simulink model "MR_CIGRE_GENERALIZADO"  (R2017b)
settings: Solver=ode23tb  StartTime=0.0  StopTime=t_sim  RelTol=1e-4
values from neighbouring files (symbols this model uses):
  BAT1_CONT = 0    [Dados_MR_CIGRE_generalizado.m]
  BAT2_CONT = 0    [Dados_MR_CIGRE_generalizado.m]
  Cdc = 19.24E-6/2    (= 9.62e-06)    [Dados_de_Intermit.m]    (also in Dados_de_Intermit_old.m)
  Cf = 5E-6    (= 5e-06)    [Dados_de_Intermit.m]    (also in Dados_de_Intermit_old.m)
  f0 = 50    [Dados_MR_CIGRE_generalizado.m]
  Imax_solar1 = 1.5 * I_nom_solar1 * sqrt(2)    [Dados_de_Intermit.m]
  Imax_solar2 = 1.5 * I_nom_solar2 * sqrt(2)    [Dados_de_Intermit.m]
  Ki_interm = (R+ron)/ti    (= 201.76)    [Dados_de_Intermit.m]
  Kp_cp = 0.2    [Dados_de_Intermit.m]
  Kp_cr = 0.4e-3    (= 0.0004)    [Dados_de_Intermit.m]
  Kp_interm = L/ti    (= 2.7)    [Dados_de_Intermit.m]
  L = 1.35E-3    (= 0.00135)    [Dados_de_Intermit.m]    (also in Dados_de_Intermit_old.m)
  LPF_P_Interm = 100    [Dados_de_Intermit.m]
  P_Solar1 = 21e3    (= 21000)    [Dados_MR_CIGRE_generalizado.m]
  P_Solar2 = 21e3    (= 21000)    [Dados_MR_CIGRE_generalizado.m]
  PQ_ref_time_bat1 = t_estab    (= 1)    [Dados_MR_CIGRE_generalizado.m]
  Pref_Bat1 = 0*1e3    (= 0)    [Dados_MR_CIGRE_generalizado.m]
  Qref_Bat1 = 0*1e3    (= 0)    [Dados_MR_CIGRE_generalizado.m]
  Qref_Solar = 0    [Dados_MR_CIGRE_generalizado.m]
  R = 0.1    [Dados_de_Intermit.m]    (also in Dados_de_Intermit_old.m)
  ron = 0.88E-3    (= 0.00088)    [Dados_de_Intermit.m]    (also in Dados_de_Intermit_old.m)
  Sb_Bat1 = 45e3    (= 45000)    [Dados_MR_CIGRE_generalizado.m]
  Sb_sol1 = 20e3    (= 20000)    [Dados_MR_CIGRE_generalizado.m]
  Sb_sol2 = 20e3    (= 20000)    [Dados_MR_CIGRE_generalizado.m]
  t_atraso = 0    [Dados_MR_CIGRE_generalizado.m]
  theta1 = 45*rad    (= 0.785398163397)    [Dados_MR_CIGRE_generalizado.m]
  theta2 = 45*rad    (= 0.785398163397)    [Dados_MR_CIGRE_generalizado.m]
  ti_cp = 10e-3    (= 0.01)    [Dados_de_Intermit.m]
  ti_cr = 10e-3    (= 0.01)    [Dados_de_Intermit.m]
  tilha = 0.6    [Dados_MR_CIGRE_generalizado.m]
  tsinc = 6    [Dados_MR_CIGRE_generalizado.m]
  Vdc = 700    [Dados_de_Intermit.m]    (also in Dados_de_Intermit_old.m)
  Vs1 = 20000    [Dados_MR_CIGRE_generalizado.m]
  Vs2 = 400    [Dados_MR_CIGRE_generalizado.m]
  w0 = 2*pi*f0    (= 314.159265359)    [Dados_MR_CIGRE_generalizado.m]
undefined symbols (not defined in the file or in its folder): Cdc_Bat1, Cf_Bat1, cont_fre, cont_ten, I_max_Bat1, Is_bat1, K_iff_Bat1, Kcij, Ki_Bat1, Kie, Kiw, Kp_Bat1, Kpe, Kpw, Kv_Bat1, Kvi_DC, Kvp_DC, L_10_18, L_12_13, L_13_14, L_14_15, L_1_2, L_2_3, L_3_11, L_3_4, L_4_12, L_4_5, L_5_6, L_6_16, L_6_7, L_7_8, L_8_9, L_9_10, L_9_17, L_Bat1, L_Bat2, L_Virt_Bat1, L_Virt_Bat2, LC_Bat2, Lfsj, LPF_Ci_Bat1, LPF_Ci_Bat2, LPF_Cv_Bat1, LPF_P_Bat1, LPF_Q_Bat1, LPF_Vdc, m_Bat1, n_Bat1, PQ_ref_taxavar_bat1, R_10_18, R_12_13, R_13_14, R_14_15, R_1_2, R_2_3, R_3_11, R_3_4, R_4_12, R_4_5, R_5_6 ... (+32)
libraries: powerlib x158, powerlib_meascontrol x59, re_lib x2, simulink x1
(part 3 of 4)

== system MR_CIGRE_GENERALIZADO/Banco de Baterias_1/Bateria e Conversor CC//CC ==
  note: Bateria
  note: Conversor CC e chopper
  note: Medidas Bateria
  D : Inport
  CM2 : powerlib/Measurements/Current Measurement  PhasorSimulation=off  OutputType=Complex  PSBequivalent=0
  DC Voltage Source : powerlib/Electrical Sources/DC Voltage Source  Amplitude=Voc_bat1  Measurements=None
  P : Product  Inputs=**
  Series RLC Branch : powerlib/Elements/Series RLC Branch  LConnTagsString=__new0  RConnTagsString=__new0  BranchType=RL  Resistance=Rfsj  Inductance=Lfsj  SetiL0=on  InitialCurrent=0  Capacitance=1e-6  Setx0=off  InitialVoltage=0  Measurements=None
  Series RLC Branch1 : powerlib/Elements/Series RLC Branch  LConnTagsString=__new0  RConnTagsString=__new0  BranchType=R  Resistance=Rb_bat1  Inductance=1e-3  SetiL0=off  InitialCurrent=0  Capacitance=1e-6  Setx0=off  InitialVoltage=0  Measurements=None
  Two-Quadrant DC/DC Converter : powerlib/Power Electronics/Two-Quadrant DC//DC Converter  ModelType=Average model (D-controlled)  Ron=1e-3  Rs=1e6  Cs=inf  Vforward=[0,0]  Ron_Diode=1e-3  Rs_Diode=1e6  Cs_Diode=inf  Vf_Diode=1e-3  Rs_CurrentSource=inf
      settings: SourceProductName=Simscape Power Systems  SourceProductBaseCode=PS
  VM2 : powerlib/Measurements/Voltage Measurement  PhasorSimulation=off  OutputType=Complex  PSBequivalent=0
  + out : PMIOPort  Port=1  Side=Left
  - out : PMIOPort  Port=2  Side=Left
  Ibat : Outport
  Vbat : Outport  Port=2
  Pbat : Outport  Port=3
  wires:
  CM2/1 -> P/2, Ibat/1
  P/1 -> Pbat/1
  VM2/1 -> P/1, Vbat/1
  D/1 -> Two-Quadrant DC/DC Converter/1
  connections:
  CM2/RConn1 -- Series RLC Branch/LConn1
  Two-Quadrant DC/DC Converter/LConn1 -- Series RLC Branch/RConn1
  Series RLC Branch1/LConn1 -- DC Voltage Source/RConn1
  CM2/LConn1 -- VM2/LConn1 -- Series RLC Branch1/RConn1
  + out/RConn1 -- Two-Quadrant DC/DC Converter/RConn1
  Two-Quadrant DC/DC Converter/RConn2 -- - out/RConn1 -- DC Voltage Source/LConn1 -- VM2/LConn2

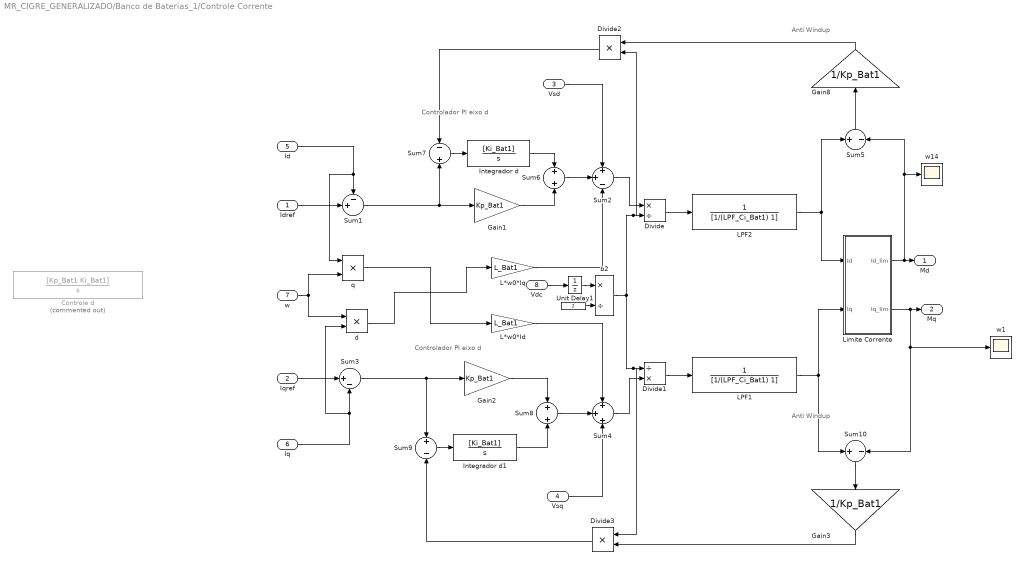
== system MR_CIGRE_GENERALIZADO/Banco de Baterias_1/Controle Corrente ==
  note: Anti Windup
  note: Controlador PI eixo d
  note: Controlador PI eixo d
  note: Anti Windup
  Idref : Inport
  Iqref : Inport  Port=2
  Vsd : Inport  Port=3
  Vsq : Inport  Port=4
  Id : Inport  Port=5
  Iq : Inport  Port=6
  w : Inport  Port=7
  Vdc : Inport  Port=8
  " " : Constant  Value=2
  Controle d : TransferFcn  Commented=on  Numerator=[Kp_Bat1 Ki_Bat1]  Denominator=[1 0]
  Divide : Product  Inputs=*/
  Divide1 : Product  Inputs=/*
  Divide2 : Product  Inputs=**
  Divide3 : Product  Inputs=**
  Gain1 : Gain  Gain=Kp_Bat1
  Gain2 : Gain  Gain=Kp_Bat1
  Gain3 : Gain  Gain=1/Kp_Bat1
  Gain8 : Gain  Gain=1/Kp_Bat1
  Integrador d : TransferFcn  Numerator=[Ki_Bat1]  Denominator=[1 0]
  Integrador d1 : TransferFcn  Numerator=[Ki_Bat1]  Denominator=[1 0]
  L*w0*Id : Gain  Gain=L_Bat1
  L*w0*Iq : Gain  Gain=L_Bat1
  LPF1 : TransferFcn  Denominator=[1/(LPF_Ci_Bat1) 1]
  LPF2 : TransferFcn  Denominator=[1/(LPF_Ci_Bat1) 1]
  Limite Corrente : Subsystem
  Sum1 : Sum  Inputs=-+|
  Sum10 : Sum  Inputs=+|-
  Sum2 : Sum  Inputs=+|+|-
  Sum3 : Sum  Inputs=|+-
  Sum4 : Sum  Inputs=+|+|+
  Sum5 : Sum  Inputs=+|-
  Sum6 : Sum  Inputs=+|+
  Sum7 : Sum  Inputs=-+
  Sum8 : Sum  Inputs=+|+
  Sum9 : Sum  Inputs=+-
  Unit Delay1 : UnitDelay  InitialCondition=800  SampleTime=5E-5
  b2 : Product  Inputs=*/
  d : Product  Inputs=**
  q : Product  Inputs=**
  w1 : Scope
  w14 : Scope
  Md : Outport
  Mq : Outport  Port=2
  wires:
  Vsd/1 -> Sum2/1
  Limite Corrente/2(Iq_lim) -> Sum10/2, w1/1, Mq/1
  Sum2/1 -> Divide/1
  Iq/1 -> d/2, Sum3/2
  Iqref/1 -> Sum3/1
  w/1 -> d/1, q/2
  q/1 -> L*w0*Id/1
  L*w0*Iq/1 -> Sum2/3
  b2/1 -> Divide2/2, Divide/2, Divide3/1, Divide1/1
  d/1 -> L*w0*Iq/1
  Idref/1 -> Sum1/2
  Sum4/1 -> Divide1/2
  Sum6/1 -> Sum2/2
  Sum8/1 -> Sum4/2
  L*w0*Id/1 -> Sum4/1
  Id/1 -> q/1, Sum1/1
  Vsq/1 -> Sum4/3
  Divide1/1 -> LPF1/1
  Divide/1 -> LPF2/1
  LPF2/1 -> Limite Corrente/1(Id), Sum5/1
  LPF1/1 -> Limite Corrente/2(Iq), Sum10/1
  Vdc/1 -> Unit Delay1/1
  " "/1 -> b2/2
  Unit Delay1/1 -> b2/1
  Limite Corrente/1(Id_lim) -> w14/1, Sum5/2, Md/1
  Sum7/1 -> Integrador d/1
  Sum1/1 -> Sum7/2, Gain1/1
  Gain1/1 -> Sum6/2
  Sum5/1 -> Gain8/1
  Integrador d/1 -> Sum6/1
  Gain8/1 -> Divide2/1
  Sum9/1 -> Integrador d1/1
  Integrador d1/1 -> Sum8/2
  Gain2/1 -> Sum8/1
  Sum3/1 -> Sum9/1, Gain2/1
  Sum10/1 -> Gain3/1
  Gain3/1 -> Divide3/2
  Divide2/1 -> Sum7/1
  Divide3/1 -> Sum9/2

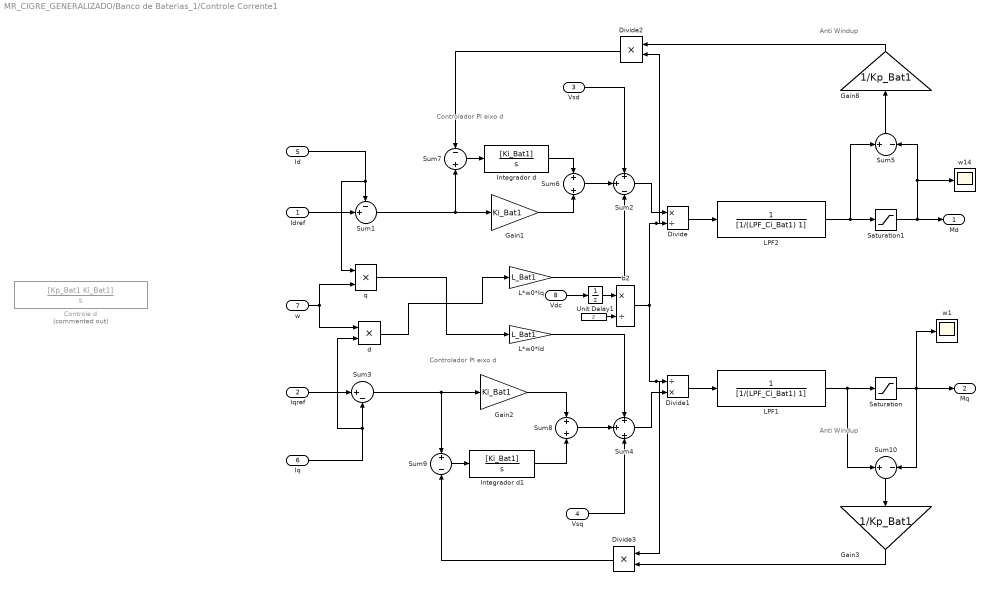
== system MR_CIGRE_GENERALIZADO/Banco de Baterias_1/Controle Corrente1 ==
  note: Anti Windup
  note: Controlador PI eixo d
  note: Controlador PI eixo d
  note: Anti Windup
  Idref : Inport
  Iqref : Inport  Port=2
  Vsd : Inport  Port=3
  Vsq : Inport  Port=4
  Id : Inport  Port=5
  Iq : Inport  Port=6
  w : Inport  Port=7
  Vdc : Inport  Port=8
  " " : Constant  Value=2
  Controle d : TransferFcn  Commented=on  Numerator=[Kp_Bat1 Ki_Bat1]  Denominator=[1 0]
  Divide : Product  Inputs=*/
  Divide1 : Product  Inputs=/*
  Divide2 : Product  Inputs=**
  Divide3 : Product  Inputs=**
  Gain1 : Gain  Gain=Ki_Bat1
  Gain2 : Gain  Gain=Ki_Bat1
  Gain3 : Gain  Gain=1/Kp_Bat1
  Gain8 : Gain  Gain=1/Kp_Bat1
  Integrador d : TransferFcn  Numerator=[Ki_Bat1]  Denominator=[1 0]
  Integrador d1 : TransferFcn  Numerator=[Ki_Bat1]  Denominator=[1 0]
  L*w0*Id : Gain  Gain=L_Bat1
  L*w0*Iq : Gain  Gain=L_Bat1
  LPF1 : TransferFcn  Denominator=[1/(LPF_Ci_Bat1) 1]
  LPF2 : TransferFcn  Denominator=[1/(LPF_Ci_Bat1) 1]
  Saturation : Saturate  UpperLimit=1  LowerLimit=-1
  Saturation1 : Saturate  UpperLimit=1  LowerLimit=-1
  Sum1 : Sum  Inputs=-+|
  Sum10 : Sum  Inputs=+|-
  Sum2 : Sum  Inputs=+|+|-
  Sum3 : Sum  Inputs=|+-
  Sum4 : Sum  Inputs=+|+|+
  Sum5 : Sum  Inputs=+|-
  Sum6 : Sum  Inputs=+|+
  Sum7 : Sum  Inputs=-+
  Sum8 : Sum  Inputs=+|+
  Sum9 : Sum  Inputs=+-
  Unit Delay1 : UnitDelay  InitialCondition=800  SampleTime=5E-5
  b2 : Product  Inputs=*/
  d : Product  Inputs=**
  q : Product  Inputs=**
  w1 : Scope
  w14 : Scope
  Md : Outport
  Mq : Outport  Port=2
  wires:
  Vsd/1 -> Sum2/1
  Saturation/1 -> Sum10/2, w1/1, Mq/1
  Sum2/1 -> Divide/1
  Iq/1 -> d/2, Sum3/2
  Iqref/1 -> Sum3/1
  w/1 -> d/1, q/2
  q/1 -> L*w0*Id/1
  L*w0*Iq/1 -> Sum2/3
  b2/1 -> Divide2/2, Divide/2, Divide3/1, Divide1/1
  d/1 -> L*w0*Iq/1
  Idref/1 -> Sum1/2
  Sum4/1 -> Divide1/2
  Sum6/1 -> Sum2/2
  Sum8/1 -> Sum4/2
  L*w0*Id/1 -> Sum4/1
  Id/1 -> q/1, Sum1/1
  Vsq/1 -> Sum4/3
  Divide1/1 -> LPF1/1
  Divide/1 -> LPF2/1
  LPF2/1 -> Sum5/1, Saturation1/1
  LPF1/1 -> Sum10/1, Saturation/1
  Vdc/1 -> Unit Delay1/1
  " "/1 -> b2/2
  Unit Delay1/1 -> b2/1
  Saturation1/1 -> Sum5/2, w14/1, Md/1
  Sum7/1 -> Integrador d/1
  Sum1/1 -> Sum7/2, Gain1/1
  Gain1/1 -> Sum6/2
  Sum5/1 -> Gain8/1
  Integrador d/1 -> Sum6/1
  Gain8/1 -> Divide2/1
  Sum9/1 -> Integrador d1/1
  Integrador d1/1 -> Sum8/2
  Gain2/1 -> Sum8/1
  Sum3/1 -> Sum9/1, Gain2/1
  Sum10/1 -> Gain3/1
  Gain3/1 -> Divide3/2
  Divide2/1 -> Sum7/1
  Divide3/1 -> Sum9/2

== system MR_CIGRE_GENERALIZADO/Banco de Baterias_1/Controle Tensao CC ==
  note: Controlador Corrente Bateria
  note: Controlador Tensao Vdc
  note: Calculo Duty Cycle
  Vdc : Inport
  Vbat : Inport  Port=2
  Ibat : Inport  Port=3
  Gain1 : Gain  Gain=Kcij/Tcij
  Gain2 : Gain  Gain=Kcij
  Gain5 : Gain  Gain=Kvi_DC
  Gain6 : Gain  Gain=Kvp_DC
  Gain8 : Gain  Gain=1/Kvp_DC
  Integrador d : TransferFcn  Denominator=[1 0]
  Integrador d1 : TransferFcn  Denominator=[1 0]
  LPF1 : TransferFcn  Commented=through  Denominator=[1/(LPF_Vdc) 1]
  Pref2 : Constant  Value=0
  Pref3 : Constant  Value=0
  Saturation1 : Saturate  UpperLimit=600  LowerLimit=-600
  Sum1 : Sum  Inputs=|+-
  Sum2 : Sum  Inputs=|+-
  Sum3 : Sum  Inputs=+|+||
  Sum4 : Sum  Inputs=+|+||
  Sum5 : Sum  Inputs=-+
  Sum6 : Sum  Inputs=-+
  Sum7 : Sum  Inputs=|-+
  Sum8 : Sum  Inputs=+-
  Transport Delay : TransportDelay  Commented=through  DelayTime=400e-6
  Unit Delay1 : UnitDelay  InitialCondition=200  SampleTime=5E-5
  Unit Delay2 : UnitDelay  InitialCondition=200  SampleTime=5E-5
  Vdc_ref : Constant  Value=Vdc_Bat1
  Vdc_ref1 : Constant  Value=Vdc_Bat1
  b2 : Product  Inputs=*/
  w1 : Scope  NumInputPorts=2
  w{2..3,11,14} (4 alike) : Scope
  w5 : Scope  NumInputPorts=2
  D : Outport
  wires:
  Integrador d/1 -> w2/1, Sum4/1
  Sum1/1 -> Gain6/1, Sum6/2
  Sum6/1 -> Gain5/1
  Gain6/1 -> Sum4/2
  Gain5/1 -> Integrador d/1
  Vdc_ref/1 -> w5/2, Sum1/1
  Sum2/1 -> Gain2/1, Sum5/2
  Gain2/1 -> Transport Delay/1
  Gain1/1 -> Integrador d1/1
  Sum5/1 -> Gain1/1
  Integrador d1/1 -> Sum3/1
  Gain8/1 -> Sum6/1
  Pref3/1 -> Sum5/1
  Sum3/1 -> [Uref], w14/1
  Vdc/1 -> Unit Delay1/1
  Ibat/1 -> w1/2, Sum2/2
  LPF1/1 -> w5/1, Sum1/2
  b2/1 -> D/1, w11/1
  [Uref] -> Sum7/1
  Sum4/1 -> Sum8/1, Saturation1/1
  [Iref] -> w1/1, Sum2/1
  Transport Delay/1 -> Sum3/2
  Vbat/1 -> Unit Delay2/1
  Sum7/1 -> b2/1
  Unit Delay1/1 -> b2/2, LPF1/1
  Saturation1/1 -> Sum8/2, [Iref]
  Sum8/1 -> Gain8/1
  Unit Delay2/1 -> Sum7/2

== system MR_CIGRE_GENERALIZADO/Banco de Baterias_1/Controle Potencia Droop ==
  Pref : Inport
  Qref : Inport  Port=2
  w_ref : Inport  Port=3
  V_ref : Inport  Port=4
  P : Inport  Port=5
  Q : Inport  Port=6
  Constant : Constant  Value=theta1
  Gain3 : Gain  Gain=m_Bat1
  Gain4 : Gain  Gain=w0
  Gain5 : Gain  Gain=n_Bat1
  Gain6 : Gain  Gain=Vs2*sqrt(2)/sqrt(3)
  Referência Fonte : MATLAB Function  TreatAsAtomicUnit=on
  Sum1 : Sum  Inputs=+-|
  Sum2 : Sum  Inputs=+-|
  Sum3 : Sum  Inputs=-+|
  Sum4 : Sum  Inputs=-+|
  pu1 : Gain  Gain=1/Sb_Bat1
  pu2 : Gain  Gain=1/Sb_Bat1
  Vref : Outport
  Wref : Outport  Port=2
  wires:
  V_ref/1 -> Sum2/1
  Sum1/1 -> Gain4/1
  Sum2/1 -> Gain6/1
  Sum3/1 -> pu1/1
  Gain6/1 -> Vref/1
  w_ref/1 -> Sum1/1
  Sum4/1 -> pu2/1
  Qref/1 -> Sum4/1
  Gain3/1 -> Sum2/2
  Gain5/1 -> Sum1/2
  Q/1 -> Sum4/2
  Pref/1 -> Sum3/1
  Gain4/1 -> Wref/1
  P/1 -> Sum3/2
  pu1/1 -> Referência Fonte/1(P)
  pu2/1 -> Referência Fonte/2(Q)
  Referência Fonte/1(Plinha) -> Gain5/1
  Referência Fonte/2(Qlinha) -> Gain3/1
  Constant/1 -> Referência Fonte/3(theta)

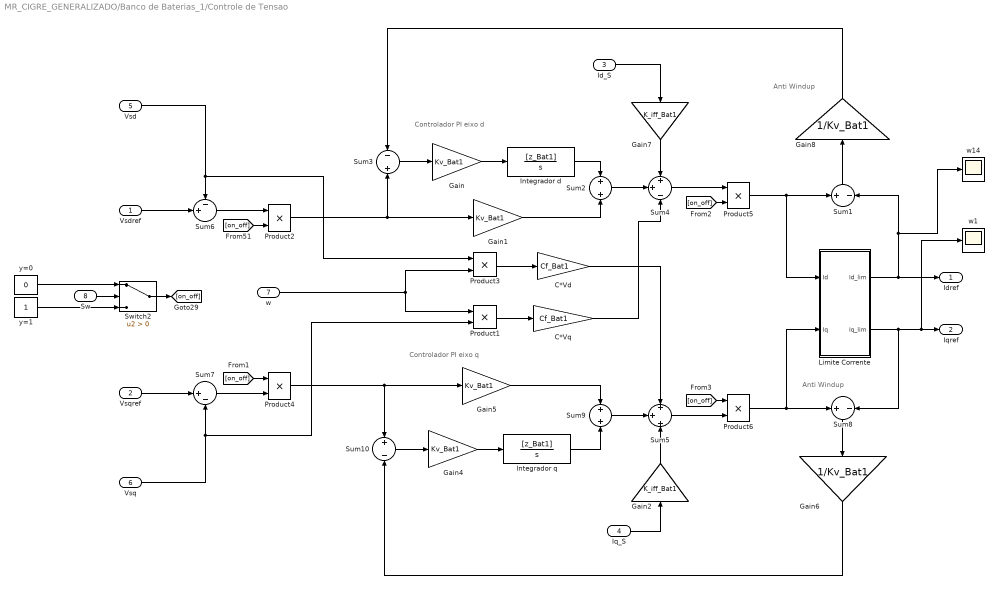
== system MR_CIGRE_GENERALIZADO/Banco de Baterias_1/Controle de Tensao ==
  note: Controlador PI eixo d
  note: Controlador PI eixo q
  note: Anti Windup
  note: Anti Windup
  Vsdref : Inport
  Vsqref : Inport  Port=2
  Id_S : Inport  Port=3
  Iq_S : Inport  Port=4
  Vsd : Inport  Port=5
  Vsq : Inport  Port=6
  w : Inport  Port=7
  Sw : Inport  Port=8
  C*Vd : Gain  Gain=Cf_Bat1
  C*Vq : Gain  Gain=Cf_Bat1
  Gain{,1,4..5} (4 alike) : Gain  Gain=Kv_Bat1
  Gain2 : Gain  Gain=K_iff_Bat1
  Gain6 : Gain  Gain=1/Kv_Bat1
  Gain7 : Gain  Gain=K_iff_Bat1
  Gain8 : Gain  Gain=1/Kv_Bat1
  Integrador d : TransferFcn  Numerator=[z_Bat1]  Denominator=[1 0]
  Integrador q : TransferFcn  Numerator=[z_Bat1]  Denominator=[1 0]
  Limite Corrente : Subsystem
  Product{1..6} (6 alike) : Product
  Sum1 : Sum  Inputs=+|-
  Sum10 : Sum  Inputs=+-
  Sum2 : Sum  Inputs=+|+
  Sum3 : Sum  Inputs=-+
  Sum4 : Sum  Inputs=+|+|-
  Sum5 : Sum  Inputs=+|+|+
  Sum6 : Sum  Inputs=-+|
  Sum7 : Sum  Inputs=|+-
  Sum8 : Sum  Inputs=+|-
  Sum9 : Sum  Inputs=+|+
  Switch2 : Switch  Criteria=u2 > Threshold
  w1 : Scope
  w14 : Scope
  y=0 : Constant  Value=0
  y=1 : Constant
  Idref : Outport
  Iqref : Outport  Port=2
  wires:
  y=1/1 -> Switch2/3
  y=0/1 -> Switch2/1
  Sw/1 -> Switch2/2
  w/1 -> Product3/2, Product1/1
  Vsd/1 -> Sum6/1, Product3/1
  Vsq/1 -> Sum7/2, Product1/2
  Product3/1 -> C*Vd/1
  C*Vq/1 -> Sum4/3
  Vsqref/1 -> Sum7/1
  Sum2/1 -> Sum4/2
  Vsdref/1 -> Sum6/2
  C*Vd/1 -> Sum5/1
  Sum7/1 -> Product4/2
  Product1/1 -> C*Vq/1
  Sum6/1 -> Product2/1
  Sum4/1 -> Product5/1
  Sum5/1 -> Product6/2
  Product5/1 -> Limite Corrente/1(Id), Sum1/1
  Limite Corrente/1(Id_lim) -> w14/1, Sum1/2, Idref/1
  Gain/1 -> Integrador d/1
  Gain1/1 -> Sum2/2
  Sum3/1 -> Gain/1
  Sum1/1 -> Gain8/1
  Gain8/1 -> Sum3/1
  Limite Corrente/2(Iq_lim) -> Sum8/2, w1/1, Iqref/1
  Sum9/1 -> Sum5/2
  Sum10/1 -> Gain4/1
  Gain4/1 -> Integrador q/1
  Integrador q/1 -> Sum9/2
  Gain5/1 -> Sum9/1
  Gain6/1 -> Sum10/2
  Sum8/1 -> Gain6/1
  Integrador d/1 -> Sum2/1
  Switch2/1 -> [on_off]
  [on_off] -> Product2/2
  [on_off] -> Product4/1
  [on_off] -> Product5/2
  [on_off] -> Product6/1
  Id_S/1 -> Gain7/1
  Gain7/1 -> Sum4/1
  Iq_S/1 -> Gain2/1
  Gain2/1 -> Sum5/3
  Product6/1 -> Limite Corrente/2(Iq), Sum8/1
  Product2/1 -> Sum3/2, Gain1/1
  Product4/1 -> Sum10/1, Gain5/1

== system MR_CIGRE_GENERALIZADO/Banco de Baterias_1/Controle de potência modo conectado ==
  Pref : Inport
  Qref : Inport  Port=2
  Vsd : Inport  Port=3
  Vsq : Inport  Port=4
  Gain : Gain  Gain=2/3
  Gain1 : Gain  Gain=2/3
  Subsystem : Subsystem  Commented=on
  Sum1 : Sum  Inputs=|++
  Sum2 : Sum  Inputs=|+-
  Sum3 : Sum  Inputs=-+|
  Sum6 : Sum  Inputs=+-|
  a{1,3..7} (6 alike) : Product  Inputs=**
  a2 : Product  Inputs=*/
  b2 : Product  Inputs=*/
  w1 : Scope
  w14 : Scope
  Irefd : Outport
  Irefq : Outport  Port=2
  wires:
  a2/1 -> Gain/1
  b2/1 -> Gain1/1
  Sum6/1 -> a2/1
  Sum1/1 -> a2/2
  a3/1 -> Sum6/2
  a1/1 -> Sum6/1
  Pref/1 -> a7/1, a1/1
  Vsd/1 -> a6/2, a4/2, a4/1, a1/2
  Vsq/1 -> a7/2, a5/1, a5/2, a3/2
  a5/1 -> Sum2/2, Sum1/1
  a4/1 -> Sum2/1, Sum1/2
  Sum3/1 -> b2/1
  Sum2/1 -> b2/2
  a7/1 -> Sum3/2
  a6/1 -> Sum3/1
  Qref/1 -> a6/1, a3/1
  Gain/1 -> w14/1, Irefd/1
  Gain1/1 -> w1/1, Irefq/1

== system MR_CIGRE_GENERALIZADO/Banco de Baterias_1/Controle wt2 ==
  Sys_wt : Inport
  Sys_w : Inport  Port=2
  w_ref : Inport  Port=3
  Sw : Inport  Port=4
  Integrator1 : Integrator  WrapState=on  WrappedStateUpperValue=2*pi()  WrappedStateLowerValue=0
  Switch2 : Switch  Criteria=u2 > Threshold
  Switch4 : Switch  Criteria=u2 > Threshold
  wt : Outport
  wires:
  Integrator1/1 -> Switch4/3
  Switch4/1 -> wt/1
  Sys_wt/1 -> Switch4/1
  Switch2/1 -> Integrator1/1
  Sw/1 -> Switch4/2, Switch2/2
  Sys_w/1 -> Switch2/1
  w_ref/1 -> Switch2/3

== system MR_CIGRE_GENERALIZADO/Banco de Baterias_1/Elo CC ==
  CM1 : powerlib/Measurements/Current Measurement  PhasorSimulation=off  OutputType=Complex  PSBequivalent=0
  CM2 : powerlib/Measurements/Current Measurement  PhasorSimulation=off  OutputType=Complex  PSBequivalent=0
  CM3 : powerlib/Measurements/Current Measurement  PhasorSimulation=off  OutputType=Complex  PSBequivalent=0
  DC Voltage Source : powerlib/Electrical Sources/DC Voltage Source  Commented=on  Amplitude=Vdc_Bat1  Measurements=None
  P : Product  Commented=on  Inputs=**
  P1 : Product  Commented=on  Inputs=**
  Parallel RLC Branch1 : powerlib/Elements/Parallel RLC Branch  LConnTagsString=a  RConnTagsString=__new0  BranchType=R  Resistance=1500  Inductance=0  SetiL0=off  InitialCurrent=0  Capacitance=Cdc_Bat1  Setx0=on  InitialVoltage=700  Measurements=None
  Parallel RLC Branch2 : powerlib/Elements/Parallel RLC Branch  LConnTagsString=a  RConnTagsString=__new0  BranchType=C  Resistance=10000000  Inductance=0  SetiL0=off  InitialCurrent=0  Capacitance=Cdc_Bat1  Setx0=on  InitialVoltage=700  Measurements=None
  Parallel RLC Branch3 : powerlib/Elements/Parallel RLC Branch  LConnTagsString=a  RConnTagsString=__new0  BranchType=R  Resistance=0.00001  Inductance=0  SetiL0=off  InitialCurrent=0  Capacitance=Cdc_Bat1  Setx0=on  InitialVoltage=700  Measurements=None
  VM1 : powerlib/Measurements/Voltage Measurement  PhasorSimulation=off  OutputType=Complex  PSBequivalent=0
  w1 : Scope  Commented=on
  w2 : Scope  Commented=on
  w3 : Scope  Commented=on  NumInputPorts=2
  w7 : Scope  Commented=on
  + in : PMIOPort  Port=1  Side=Left
  - in : PMIOPort  Port=2  Side=Left
  + out : PMIOPort  Port=3  Side=Right
  - out : PMIOPort  Port=4  Side=Right
  Vdc : Outport
  wires:
  P/1 -> w3/2, w2/1
  CM1/1 -> P/1
  CM2/1 -> w7/1
  P1/1 -> w3/1, w1/1
  CM3/1 -> P1/1
  VM1/1 -> Vdc/1, P1/2, P/2
  connections:
  Parallel RLC Branch2/LConn1 -- CM2/LConn1
  CM2/RConn1 -- Parallel RLC Branch3/LConn1 -- VM1/LConn1 -- CM1/LConn1
  - in/RConn1 -- Parallel RLC Branch1/RConn1 -- - out/RConn1 -- DC Voltage Source/LConn1 -- VM1/LConn2 -- Parallel RLC Branch2/RConn1
  Parallel RLC Branch1/LConn1 -- CM3/LConn1 -- + in/RConn1
  DC Voltage Source/RConn1 -- CM1/RConn1 -- + out/RConn1
  CM3/RConn1 -- Parallel RLC Branch3/RConn1

== system MR_CIGRE_GENERALIZADO/Banco de Baterias_1/Imp. Virtual1 ==
  Id : Inport
  Iq : Inport  Port=2
  W : Inport  Port=3
  HPF1 : TransferFcn  Numerator=[1 0]  Denominator=[1 100]
  HPF2 : TransferFcn  Numerator=[1 0]  Denominator=[1 100]
  Product1 : Product
  Product3 : Product
  Sum1 : Sum  Inputs=|++
  Sum2 : Sum  Inputs=|++
  Sum5 : Sum  Inputs=++|
  Sum6 : Sum  Inputs=++|
  Zvdd : Gain  Gain=L_Virt_Bat1
  Zvdq1 : Gain  Gain=-L_Virt_Bat1
  Zvqd : Gain  Gain=L_Virt_Bat1
  Zvqq : Gain  Gain=L_Virt_Bat1
  Zvqq1 : Gain  Gain=R_Virt_Bat1
  Zvqq2 : Gain  Gain=R_Virt_Bat1
  Vd_Zv : Outport
  Vq_Zv : Outport  Port=2
  wires:
  Zvqd/1 -> Product3/2
  W/1 -> Product1/2, Product3/1
  Sum6/1 -> Vq_Zv/1
  Zvdd/1 -> HPF1/1
  Product1/1 -> Sum5/2
  Zvqq/1 -> HPF2/1
  Id/1 -> Zvqd/1, Zvqq2/1, Zvdd/1
  Product3/1 -> Sum6/1
  Sum5/1 -> Vd_Zv/1
  Zvdq1/1 -> Product1/1
  Iq/1 -> Zvqq1/1, Zvdq1/1, Zvqq/1
  HPF2/1 -> Sum1/1
  Zvqq1/1 -> Sum1/2
  Sum1/1 -> Sum6/2
  HPF1/1 -> Sum2/1
  Zvqq2/1 -> Sum2/2
  Sum2/1 -> Sum5/1

== system MR_CIGRE_GENERALIZADO/Banco de Baterias_1/Inversor CC//CA ==
  Vabc : Inport
  R+ron+L VSC2 : powerlib/Elements/Three-Phase Series RLC Branch  LConnTagsString=A|B|C  RConnTagsString=A|B|C  BranchType=RL  Resistance=R_Bat1+ron_Bat1  Inductance=L_Bat1  Capacitance=1e-6  Measurements=None
  Sequence Analyzer5 : powerlib_meascontrol/Measurements/Sequence Analyzer  Commented=on  Freq=60  n=1  seq=Positive  InInit=[1, 0]  Ts=0
      settings: SourceProductName=Simscape Power Systems  SourceProductBaseCode=PS
  Three-Phase Series RLC Branch1 : powerlib/Elements/Three-Phase Series RLC Branch  LConnTagsString=A|B|C  RConnTagsString=A|B|C  BranchType=C  Resistance=1  Inductance=1e-3  Capacitance=Cf_Bat1  Measurements=None
  V&I - VSC2 2 : powerlib/Measurements/Three-Phase V-I Measurement  VoltageMeasurement=phase-to-ground  SetLabelV=off  LabelV=Vabc  Vpu=off  VpuLL=off  CurrentMeasurement=yes  SetLabelI=off  LabelI=Iabc  Ipu=off  Pbase=100e6  Vbase=500e3  OutputType=Complex  PhasorSimulation=off  PSBequivalent=0
  VSC (Average Model) : powerlib/Power Electronics/Universal Bridge  Arms=3  SnubberResistance=1e5  SnubberCapacitance=inf  Device=Average-model based VSC  Ron=1e-3  Lon=0  ForwardVoltages="[  0  0  ]"  ForwardVoltage=0  GTOparameters=[ 10e-6 , 20e-6 ]  IGBTparameters=[ 1e-6 , 2e-6 ]  Measurements=None  Measurements_2=None  converterType=Rectifier
  w4 : Scope  Commented=on
  Va : PMIOPort  Port=1  Side=Right
  Vb : PMIOPort  Port=2  Side=Right
  Vc : PMIOPort  Port=3  Side=Right
  GND : PMIOPort  Port=4  Side=Right
  + : PMIOPort  Port=5  Side=Left
  - : PMIOPort  Port=6  Side=Left
  Vabc_M : Outport
  Iabc_M : Outport  Port=2
  wires:
  V&I - VSC2 2/2 -> Iabc_M/1
  Sequence Analyzer5/1 -> w4/1
  V&I - VSC2 2/1 -> Vabc_M/1
  Vabc/1 -> Sequence Analyzer5/1, VSC (Average Model)/1
  connections:
  Three-Phase Series RLC Branch1/RConn1 -- Three-Phase Series RLC Branch1/RConn3 -- Three-Phase Series RLC Branch1/RConn2 -- GND/RConn1
  V&I - VSC2 2/RConn1 -- R+ron+L VSC2/LConn1
  V&I - VSC2 2/RConn2 -- R+ron+L VSC2/LConn2
  V&I - VSC2 2/RConn3 -- R+ron+L VSC2/LConn3
  Three-Phase Series RLC Branch1/LConn1 -- Va/RConn1 -- R+ron+L VSC2/RConn1
  Three-Phase Series RLC Branch1/LConn2 -- Vb/RConn1 -- R+ron+L VSC2/RConn2
  Three-Phase Series RLC Branch1/LConn3 -- Vc/RConn1 -- R+ron+L VSC2/RConn3
  VSC (Average Model)/LConn1 -- V&I - VSC2 2/LConn1
  VSC (Average Model)/LConn2 -- V&I - VSC2 2/LConn2
  VSC (Average Model)/LConn3 -- V&I - VSC2 2/LConn3
  VSC (Average Model)/RConn2 -- -/RConn1
  +/RConn1 -- VSC (Average Model)/RConn1

== system MR_CIGRE_GENERALIZADO/Banco de Baterias_1/Medidor de pot ==
  Vd : Inport
  Vq : Inport  Port=2
  Id : Inport  Port=3
  Iq : Inport  Port=4
  Gain : Gain  Gain=1.5
  Gain1 : Gain  Gain=1.5
  Sum1 : Sum  Inputs=+|+
  Sum2 : Sum  Inputs=-|+
  a : Product  Inputs=**
  a1 : Product  Inputs=**
  b1 : Product  Inputs=**
  b2 : Product  Inputs=**
  P : Outport
  Q : Outport  Port=2
  wires:
  a1/1 -> Sum1/2
  Vq/1 -> b2/2, a1/1
  a/1 -> Sum1/1
  b1/1 -> Sum2/1
  Sum1/1 -> Gain/1
  b2/1 -> Sum2/2
  Iq/1 -> b1/2, a1/2
  Vd/1 -> b1/1, a/1
  Id/1 -> b2/1, a/2
  Sum2/1 -> Gain1/1
  Gain/1 -> P/1
  Gain1/1 -> Q/1

== system MR_CIGRE_GENERALIZADO/Banco de Baterias_1/PLL e Medidor1 ==
  note: Medida de w e wt do Sistema
  note: Medida Vd, Vq, Iq e Id
  Iabc_M : Inport
  Iabc_S : Inport  Port=2
  Vabc_S : Inport  Port=3
  wt : Inport  Port=4
  2*pi()*f : Gain  Gain=2*pi()
  Iabc-Idq : powerlib_meascontrol/Transformations/abc to dq0  Alignment=90 degrees behind phase A axis
  Iabc-Idq1 : powerlib_meascontrol/Transformations/abc to dq0  Alignment=90 degrees behind phase A axis
  Iabc-Idq2 : powerlib_meascontrol/Transformations/abc to dq0  Alignment=90 degrees behind phase A axis
  PLL (3ph) : powerlib_meascontrol/PLL/PLL (3ph)  Fmin=1  Par_Init="[0  f0]"  ParK=[180, 3200, 1]  TcD=5E-5  MaxRateChangeFreq=120  FilterCutOffFreq=25  Ts=5E-5  AGC=on
  w8 : Scope
  Sys_wt : Outport
  Sys_w : Outport  Port=2
  Vdq0_S : Outport  Port=3
  Idq_M : Outport  Port=4
  Idq0_S : Outport  Port=5
  wires:
  PLL (3ph)/1 -> 2*pi()*f/1
  Iabc_S/1 -> Iabc-Idq/1
  Vabc_S/1 -> Iabc-Idq1/1, PLL (3ph)/1
  Iabc_M/1 -> Iabc-Idq2/1
  Iabc-Idq/1 -> Idq0_S/1
  Iabc-Idq2/1 -> Idq_M/1
  Iabc-Idq1/1 -> Vdq0_S/1
  2*pi()*f/1 -> Sys_w/1
  wt/1 -> [wt]
  PLL (3ph)/2 -> w8/1, Sys_wt/1
  [wt] -> Iabc-Idq2/2
  [wt] -> Iabc-Idq/2
  [wt] -> Iabc-Idq1/2

== system MR_CIGRE_GENERALIZADO/Banco de Baterias_1/Referecia Tensao e Freq. angular ==
  Inc_w_pu : Inport
  Inc_E_pu : Inport  Port=2
  Sum1 : Sum  Inputs=+|+
  Sum2 : Sum  Inputs=+|+
  ref : Step  Time=0  SampleTime=0
  ref2 : Step  Time=0  SampleTime=0
  w_ref_pu : Outport
  V_ref_pu : Outport  Port=2
  wires:
  Inc_E_pu/1 -> Sum1/1
  Sum1/1 -> V_ref_pu/1
  Sum2/1 -> w_ref_pu/1
  ref/1 -> Sum2/1
  Inc_w_pu/1 -> Sum2/2
  ref2/1 -> Sum1/2

== system MR_CIGRE_GENERALIZADO/Banco de Baterias_1/Referencia de  Corrente ==
  Id_feed : Inport
  Iq_feed : Inport  Port=2
  Sw_Mode : Inport  Port=3
  Id_supp : Inport  Port=4
  Iq_supp : Inport  Port=5
  LPF2 : TransferFcn  Denominator=[1/(LPF_Cv_Bat1) 1]
  LPF4 : TransferFcn  Denominator=[1/(LPF_Cv_Bat1) 1]
  Switch : Switch  Criteria=u2 > Threshold
  Switch1 : Switch  Criteria=u2 > Threshold
  Id_ref : Outport
  Iq_ref : Outport  Port=2
  wires:
  Sw_Mode/1 -> Switch/2, Switch1/2
  Switch/1 -> LPF4/1
  Switch1/1 -> LPF2/1
  Id_feed/1 -> Switch/1
  Id_supp/1 -> Switch/3
  Iq_feed/1 -> Switch1/1
  Iq_supp/1 -> Switch1/3
  LPF2/1 -> Iq_ref/1
  LPF4/1 -> Id_ref/1

== system MR_CIGRE_GENERALIZADO/Banco de Baterias_1/Referência de Potencia ==
  note: Mudança de referência: no sincronismo (sinc=1)
  note: Ref. Potencia em rampa p.u.
  sinc : Inport
  Pref_bat : Inport  Port=2
  Qref_bat : Inport  Port=3
  Pgd : Inport  Port=4
  Qgd : Inport  Port=5
  Data Store Memory : DataStoreMemory  DataStoreName=Qr  ReadBeforeWriteMsg=warning  WriteAfterWriteMsg=warning  WriteAfterReadMsg=warning  ShowAdditionalParam=off  OutDataTypeStr=double
  Data Store Memory1 : DataStoreMemory  DataStoreName=Pr  ReadBeforeWriteMsg=warning  WriteAfterWriteMsg=warning  WriteAfterReadMsg=warning  VectorParams1D=off  ShowAdditionalParam=off  OutDataTypeStr=double
  Product1 : Product
  Product2 : Product
  Rate Limiter : RateLimiter  RisingSlewLimit=PQ_ref_taxavar_bat1*Sb_Bat1  FallingSlewLimit=-PQ_ref_taxavar_bat1*Sb_Bat1  SampleTimeMode=inherited
  Rate Limiter1 : RateLimiter  RisingSlewLimit=PQ_ref_taxavar_bat1*Sb_Bat1  FallingSlewLimit=-PQ_ref_taxavar_bat1*Sb_Bat1  SampleTimeMode=inherited
  Referência Fonte : MATLAB Function  TreatAsAtomicUnit=on
  Time_init_ref : Step  Time=PQ_ref_time_bat1  SampleTime=0
  Prefbat : Outport
  Qrefbat : Outport  Port=2
  wires:
  Referência Fonte/1(Prefbat) -> Prefbat/1
  Referência Fonte/2(Qrefbat) -> Qrefbat/1
  sinc/1 -> Referência Fonte/5(sinc)
  Pgd/1 -> Referência Fonte/3(p)
  Qgd/1 -> Referência Fonte/4(q)
  Product2/1 -> Rate Limiter1/1
  Time_init_ref/1 -> Product1/2, Product2/1
  Qref_bat/1 -> Product2/2
  Product1/1 -> Rate Limiter/1
  Pref_bat/1 -> Product1/1
  Rate Limiter/1 -> Referência Fonte/1(Pref_bat)
  Rate Limiter1/1 -> Referência Fonte/2(Qref_bat)

== system MR_CIGRE_GENERALIZADO/Banco de Baterias_2/Bateria e Conversor CC//CC1 ==
  note: Bateria
  note: Conversor CC e chopper
  note: Medidas Bateria
  D : Inport
  CM2 : powerlib/Measurements/Current Measurement  PhasorSimulation=off  OutputType=Complex  PSBequivalent=0
  DC Voltage Source : powerlib/Electrical Sources/DC Voltage Source  Amplitude=Voc_bat1  Measurements=None
  P : Product  Inputs=**
  Series RLC Branch : powerlib/Elements/Series RLC Branch  LConnTagsString=__new0  RConnTagsString=__new0  BranchType=RL  Resistance=Rfsj  Inductance=Lfsj  SetiL0=on  InitialCurrent=0  Capacitance=1e-6  Setx0=off  InitialVoltage=0  Measurements=None
  Series RLC Branch1 : powerlib/Elements/Series RLC Branch  LConnTagsString=__new0  RConnTagsString=__new0  BranchType=R  Resistance=Rb_bat1  Inductance=1e-3  SetiL0=off  InitialCurrent=0  Capacitance=1e-6  Setx0=off  InitialVoltage=0  Measurements=None
  Two-Quadrant DC/DC Converter : powerlib/Power Electronics/Two-Quadrant DC//DC Converter  ModelType=Average model (D-controlled)  Ron=1e-3  Rs=1e6  Cs=inf  Vforward=[0,0]  Ron_Diode=1e-3  Rs_Diode=1e6  Cs_Diode=inf  Vf_Diode=1e-3  Rs_CurrentSource=inf
      settings: SourceProductName=Simscape Power Systems  SourceProductBaseCode=PS
  VM2 : powerlib/Measurements/Voltage Measurement  PhasorSimulation=off  OutputType=Complex  PSBequivalent=0
  + out : PMIOPort  Port=1  Side=Left
  - out : PMIOPort  Port=2  Side=Left
  Ibat : Outport
  Vbat : Outport  Port=2
  Pbat : Outport  Port=3
  wires:
  CM2/1 -> P/2, Ibat/1
  P/1 -> Pbat/1
  VM2/1 -> P/1, Vbat/1
  D/1 -> Two-Quadrant DC/DC Converter/1
  connections:
  CM2/RConn1 -- Series RLC Branch/LConn1
  Two-Quadrant DC/DC Converter/LConn1 -- Series RLC Branch/RConn1
  Series RLC Branch1/LConn1 -- DC Voltage Source/RConn1
  CM2/LConn1 -- VM2/LConn1 -- Series RLC Branch1/RConn1
  + out/RConn1 -- Two-Quadrant DC/DC Converter/RConn1
  Two-Quadrant DC/DC Converter/RConn2 -- - out/RConn1 -- DC Voltage Source/LConn1 -- VM2/LConn2

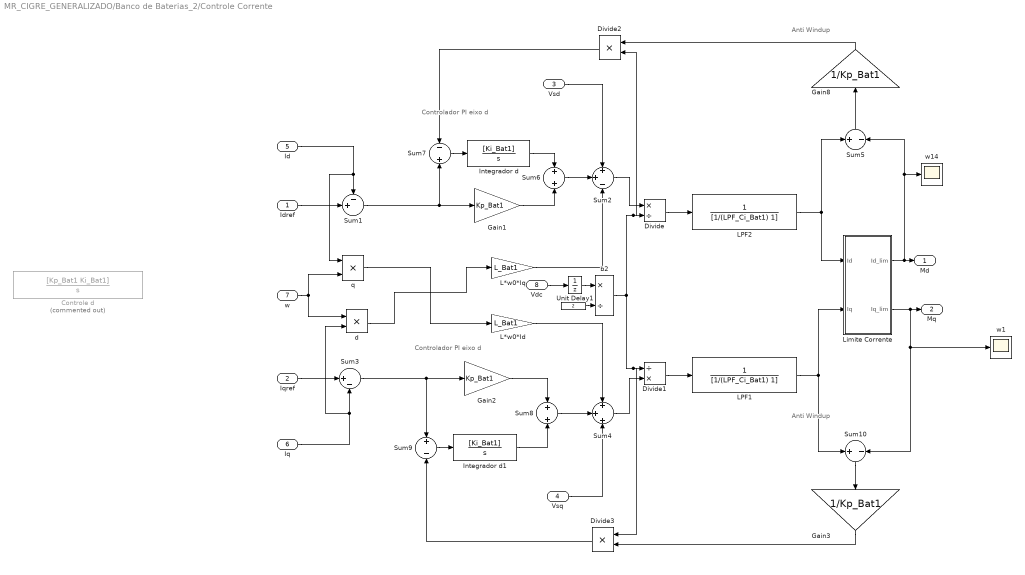
== system MR_CIGRE_GENERALIZADO/Banco de Baterias_2/Controle Corrente ==
  note: Anti Windup
  note: Controlador PI eixo d
  note: Controlador PI eixo d
  note: Anti Windup
  Idref : Inport
  Iqref : Inport  Port=2
  Vsd : Inport  Port=3
  Vsq : Inport  Port=4
  Id : Inport  Port=5
  Iq : Inport  Port=6
  w : Inport  Port=7
  Vdc : Inport  Port=8
  " " : Constant  Value=2
  Controle d : TransferFcn  Commented=on  Numerator=[Kp_Bat1 Ki_Bat1]  Denominator=[1 0]
  Divide : Product  Inputs=*/
  Divide1 : Product  Inputs=/*
  Divide2 : Product  Inputs=**
  Divide3 : Product  Inputs=**
  Gain1 : Gain  Gain=Kp_Bat1
  Gain2 : Gain  Gain=Kp_Bat1
  Gain3 : Gain  Gain=1/Kp_Bat1
  Gain8 : Gain  Gain=1/Kp_Bat1
  Integrador d : TransferFcn  Numerator=[Ki_Bat1]  Denominator=[1 0]
  Integrador d1 : TransferFcn  Numerator=[Ki_Bat1]  Denominator=[1 0]
  L*w0*Id : Gain  Gain=L_Bat1
  L*w0*Iq : Gain  Gain=L_Bat1
  LPF1 : TransferFcn  Denominator=[1/(LPF_Ci_Bat1) 1]
  LPF2 : TransferFcn  Denominator=[1/(LPF_Ci_Bat1) 1]
  Limite Corrente : Subsystem
  Sum1 : Sum  Inputs=-+|
  Sum10 : Sum  Inputs=+|-
  Sum2 : Sum  Inputs=+|+|-
  Sum3 : Sum  Inputs=|+-
  Sum4 : Sum  Inputs=+|+|+
  Sum5 : Sum  Inputs=+|-
  Sum6 : Sum  Inputs=+|+
  Sum7 : Sum  Inputs=-+
  Sum8 : Sum  Inputs=+|+
  Sum9 : Sum  Inputs=+-
  Unit Delay1 : UnitDelay  InitialCondition=800  SampleTime=5E-5
  b2 : Product  Inputs=*/
  d : Product  Inputs=**
  q : Product  Inputs=**
  w1 : Scope
  w14 : Scope
  Md : Outport
  Mq : Outport  Port=2
  wires:
  Vsd/1 -> Sum2/1
  Limite Corrente/2(Iq_lim) -> Sum10/2, w1/1, Mq/1
  Sum2/1 -> Divide/1
  Iq/1 -> d/2, Sum3/2
  Iqref/1 -> Sum3/1
  w/1 -> d/1, q/2
  q/1 -> L*w0*Id/1
  L*w0*Iq/1 -> Sum2/3
  b2/1 -> Divide2/2, Divide/2, Divide3/1, Divide1/1
  d/1 -> L*w0*Iq/1
  Idref/1 -> Sum1/2
  Sum4/1 -> Divide1/2
  Sum6/1 -> Sum2/2
  Sum8/1 -> Sum4/2
  L*w0*Id/1 -> Sum4/1
  Id/1 -> q/1, Sum1/1
  Vsq/1 -> Sum4/3
  Divide1/1 -> LPF1/1
  Divide/1 -> LPF2/1
  LPF2/1 -> Limite Corrente/1(Id), Sum5/1
  LPF1/1 -> Limite Corrente/2(Iq), Sum10/1
  Vdc/1 -> Unit Delay1/1
  " "/1 -> b2/2
  Unit Delay1/1 -> b2/1
  Limite Corrente/1(Id_lim) -> w14/1, Sum5/2, Md/1
  Sum7/1 -> Integrador d/1
  Sum1/1 -> Sum7/2, Gain1/1
  Gain1/1 -> Sum6/2
  Sum5/1 -> Gain8/1
  Integrador d/1 -> Sum6/1
  Gain8/1 -> Divide2/1
  Sum9/1 -> Integrador d1/1
  Integrador d1/1 -> Sum8/2
  Gain2/1 -> Sum8/1
  Sum3/1 -> Sum9/1, Gain2/1
  Sum10/1 -> Gain3/1
  Gain3/1 -> Divide3/2
  Divide2/1 -> Sum7/1
  Divide3/1 -> Sum9/2

== system MR_CIGRE_GENERALIZADO/Banco de Baterias_2/Controle Tensao CC1 ==
  note: Controlador Corrente Bateria
  note: Controlador Tensao Vdc
  note: Calculo Duty Cycle
  Vdc : Inport
  Vbat : Inport  Port=2
  Ibat : Inport  Port=3
  Gain1 : Gain  Gain=Kcij/Tcij
  Gain2 : Gain  Gain=Kcij
  Gain5 : Gain  Gain=Kvi_DC
  Gain6 : Gain  Gain=Kvp_DC
  Gain8 : Gain  Gain=1/Kvp_DC
  Integrador d : TransferFcn  Denominator=[1 0]
  Integrador d1 : TransferFcn  Denominator=[1 0]
  LPF1 : TransferFcn  Commented=through  Denominator=[1/(LPF_Vdc) 1]
  Pref2 : Constant  Value=0
  Pref3 : Constant  Value=0
  Saturation1 : Saturate  UpperLimit=600  LowerLimit=-600
  Sum1 : Sum  Inputs=|+-
  Sum2 : Sum  Inputs=|+-
  Sum3 : Sum  Inputs=+|+||
  Sum4 : Sum  Inputs=+|+||
  Sum5 : Sum  Inputs=-+
  Sum6 : Sum  Inputs=-+
  Sum7 : Sum  Inputs=|-+
  Sum8 : Sum  Inputs=+-
  Transport Delay : TransportDelay  Commented=through  DelayTime=400e-6
  Unit Delay1 : UnitDelay  InitialCondition=800  SampleTime=5E-5
  Unit Delay2 : UnitDelay  InitialCondition=200  SampleTime=5E-5
  Vdc_ref : Constant  Value=Vdc_Bat1
  Vdc_ref1 : Constant  Value=Vdc_Bat1
  b2 : Product  Inputs=*/
  w1 : Scope  NumInputPorts=2
  w{2..3,11,14} (4 alike) : Scope
  w5 : Scope  NumInputPorts=2
  D : Outport
  wires:
  Integrador d/1 -> w2/1, Sum4/1
  Sum1/1 -> Gain6/1, Sum6/2
  Sum6/1 -> Gain5/1
  Gain6/1 -> Sum4/2
  Gain5/1 -> Integrador d/1
  Vdc_ref/1 -> w5/2, Sum1/1
  Sum2/1 -> Gain2/1, Sum5/2
  Gain2/1 -> Transport Delay/1
  Gain1/1 -> Integrador d1/1
  Sum5/1 -> Gain1/1
  Integrador d1/1 -> Sum3/1
  Gain8/1 -> Sum6/1
  Pref3/1 -> Sum5/1
  Sum3/1 -> [Uref], w14/1
  Vdc/1 -> Unit Delay1/1
  Ibat/1 -> w1/2, Sum2/2
  LPF1/1 -> w5/1, Sum1/2
  b2/1 -> D/1, w11/1
  [Uref] -> Sum7/1
  Sum4/1 -> Sum8/1, Saturation1/1
  [Iref] -> w1/1, Sum2/1
  Transport Delay/1 -> Sum3/2
  Vbat/1 -> Unit Delay2/1
  Sum7/1 -> b2/1
  Unit Delay1/1 -> b2/2, LPF1/1
  Saturation1/1 -> Sum8/2, [Iref]
  Sum8/1 -> Gain8/1
  Unit Delay2/1 -> Sum7/2

== system MR_CIGRE_GENERALIZADO/Banco de Baterias_2/Controle Potencia Droop ==
  Pref : Inport
  Qref : Inport  Port=2
  w_ref : Inport  Port=3
  V_ref : Inport  Port=4
  P : Inport  Port=5
  Q : Inport  Port=6
  Constant : Constant  Value=theta2
  Gain3 : Gain  Gain=m_Bat1
  Gain4 : Gain  Gain=w0
  Gain5 : Gain  Gain=n_Bat1
  Gain6 : Gain  Gain=Vs2*sqrt(2)/sqrt(3)
  Referência Fonte : MATLAB Function  TreatAsAtomicUnit=on
  Sum1 : Sum  Inputs=+-|
  Sum2 : Sum  Inputs=+-|
  Sum3 : Sum  Inputs=-+|
  Sum4 : Sum  Inputs=-+|
  pu1 : Gain  Gain=1/Sb_Bat1
  pu2 : Gain  Gain=1/Sb_Bat1
  Vref : Outport
  Wref : Outport  Port=2
  wires:
  V_ref/1 -> Sum2/1
  Sum1/1 -> Gain4/1
  Sum2/1 -> Gain6/1
  Sum3/1 -> pu1/1
  Gain6/1 -> Vref/1
  w_ref/1 -> Sum1/1
  Sum4/1 -> pu2/1
  Qref/1 -> Sum4/1
  Gain3/1 -> Sum2/2
  Gain5/1 -> Sum1/2
  Q/1 -> Sum4/2
  Pref/1 -> Sum3/1
  Gain4/1 -> Wref/1
  P/1 -> Sum3/2
  pu1/1 -> Referência Fonte/1(P)
  pu2/1 -> Referência Fonte/2(Q)
  Referência Fonte/1(Plinha) -> Gain5/1
  Referência Fonte/2(Qlinha) -> Gain3/1
  Constant/1 -> Referência Fonte/3(theta)

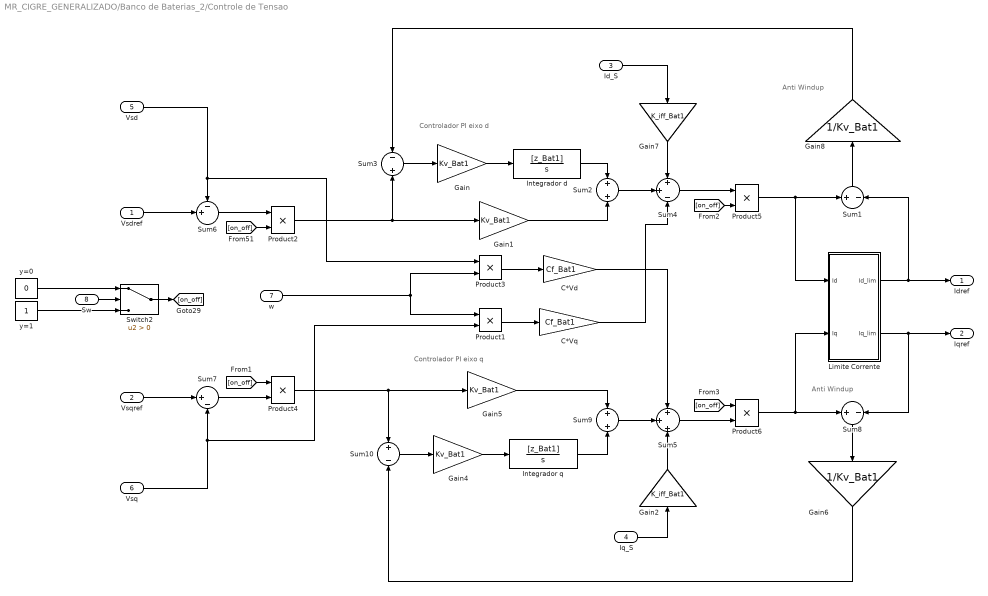
== system MR_CIGRE_GENERALIZADO/Banco de Baterias_2/Controle de Tensao ==
  note: Controlador PI eixo d
  note: Controlador PI eixo q
  note: Anti Windup
  note: Anti Windup
  Vsdref : Inport
  Vsqref : Inport  Port=2
  Id_S : Inport  Port=3
  Iq_S : Inport  Port=4
  Vsd : Inport  Port=5
  Vsq : Inport  Port=6
  w : Inport  Port=7
  Sw : Inport  Port=8
  C*Vd : Gain  Gain=Cf_Bat1
  C*Vq : Gain  Gain=Cf_Bat1
  Gain{,1,4..5} (4 alike) : Gain  Gain=Kv_Bat1
  Gain2 : Gain  Gain=K_iff_Bat1
  Gain6 : Gain  Gain=1/Kv_Bat1
  Gain7 : Gain  Gain=K_iff_Bat1
  Gain8 : Gain  Gain=1/Kv_Bat1
  Integrador d : TransferFcn  Numerator=[z_Bat1]  Denominator=[1 0]
  Integrador q : TransferFcn  Numerator=[z_Bat1]  Denominator=[1 0]
  Limite Corrente : Subsystem
  Product{1..6} (6 alike) : Product
  Sum1 : Sum  Inputs=+|-
  Sum10 : Sum  Inputs=+-
  Sum2 : Sum  Inputs=+|+
  Sum3 : Sum  Inputs=-+
  Sum4 : Sum  Inputs=+|+|-
  Sum5 : Sum  Inputs=+|+|+
  Sum6 : Sum  Inputs=-+|
  Sum7 : Sum  Inputs=|+-
  Sum8 : Sum  Inputs=+|-
  Sum9 : Sum  Inputs=+|+
  Switch2 : Switch  Criteria=u2 > Threshold
  y=0 : Constant  Value=0
  y=1 : Constant
  Idref : Outport
  Iqref : Outport  Port=2
  wires:
  y=1/1 -> Switch2/3
  y=0/1 -> Switch2/1
  Sw/1 -> Switch2/2
  w/1 -> Product3/2, Product1/1
  Vsd/1 -> Sum6/1, Product3/1
  Vsq/1 -> Sum7/2, Product1/2
  Product3/1 -> C*Vd/1
  C*Vq/1 -> Sum4/3
  Vsqref/1 -> Sum7/1
  Sum2/1 -> Sum4/2
  Vsdref/1 -> Sum6/2
  C*Vd/1 -> Sum5/1
  Sum7/1 -> Product4/2
  Product1/1 -> C*Vq/1
  Sum6/1 -> Product2/1
  Sum4/1 -> Product5/1
  Sum5/1 -> Product6/2
  Product5/1 -> Limite Corrente/1(Id), Sum1/1
  Limite Corrente/1(Id_lim) -> Sum1/2, Idref/1
  Gain/1 -> Integrador d/1
  Gain1/1 -> Sum2/2
  Sum3/1 -> Gain/1
  Sum1/1 -> Gain8/1
  Gain8/1 -> Sum3/1
  Limite Corrente/2(Iq_lim) -> Sum8/2, Iqref/1
  Sum9/1 -> Sum5/2
  Sum10/1 -> Gain4/1
  Gain4/1 -> Integrador q/1
  Integrador q/1 -> Sum9/2
  Gain5/1 -> Sum9/1
  Gain6/1 -> Sum10/2
  Sum8/1 -> Gain6/1
  Integrador d/1 -> Sum2/1
  Switch2/1 -> [on_off]
  [on_off] -> Product2/2
  [on_off] -> Product4/1
  [on_off] -> Product5/2
  [on_off] -> Product6/1
  Id_S/1 -> Gain7/1
  Gain7/1 -> Sum4/1
  Iq_S/1 -> Gain2/1
  Gain2/1 -> Sum5/3
  Product6/1 -> Limite Corrente/2(Iq), Sum8/1
  Product2/1 -> Sum3/2, Gain1/1
  Product4/1 -> Sum10/1, Gain5/1

== system MR_CIGRE_GENERALIZADO/Banco de Baterias_2/Controle de potência modo conectado ==
  Pref : Inport
  Qref : Inport  Port=2
  Vsd : Inport  Port=3
  Vsq : Inport  Port=4
  Gain : Gain  Gain=2/3
  Gain1 : Gain  Gain=2/3
  Subsystem : Subsystem  Commented=on
  Sum1 : Sum  Inputs=|++
  Sum2 : Sum  Inputs=|+-
  Sum3 : Sum  Inputs=-+|
  Sum6 : Sum  Inputs=+-|
  a{1,3..7} (6 alike) : Product  Inputs=**
  a2 : Product  Inputs=*/
  b2 : Product  Inputs=*/
  Irefd : Outport
  Irefq : Outport  Port=2
  wires:
  a2/1 -> Gain/1
  b2/1 -> Gain1/1
  Sum6/1 -> a2/1
  Sum1/1 -> a2/2
  a3/1 -> Sum6/2
  a1/1 -> Sum6/1
  Pref/1 -> a7/1, a1/1
  Vsd/1 -> a6/2, a4/2, a4/1, a1/2
  Vsq/1 -> a7/2, a5/1, a5/2, a3/2
  a5/1 -> Sum2/2, Sum1/1
  a4/1 -> Sum2/1, Sum1/2
  Sum3/1 -> b2/1
  Sum2/1 -> b2/2
  a7/1 -> Sum3/2
  a6/1 -> Sum3/1
  Qref/1 -> a6/1, a3/1
  Gain/1 -> Irefd/1
  Gain1/1 -> Irefq/1

== system MR_CIGRE_GENERALIZADO/Banco de Baterias_2/Controle wt2 ==
  Sys_wt : Inport
  Sys_w : Inport  Port=2
  w_ref : Inport  Port=3
  Sw : Inport  Port=4
  Integrator1 : Integrator  WrapState=on  WrappedStateUpperValue=2*pi()  WrappedStateLowerValue=0
  Switch2 : Switch  Criteria=u2 > Threshold
  Switch4 : Switch  Criteria=u2 > Threshold
  wt : Outport
  wires:
  Integrator1/1 -> Switch4/3
  Switch4/1 -> wt/1
  Sys_wt/1 -> Switch4/1
  Switch2/1 -> Integrator1/1
  Sw/1 -> Switch4/2, Switch2/2
  Sys_w/1 -> Switch2/1
  w_ref/1 -> Switch2/3

== system MR_CIGRE_GENERALIZADO/Banco de Baterias_2/Elo CC ==
  CM1 : powerlib/Measurements/Current Measurement  PhasorSimulation=off  OutputType=Complex  PSBequivalent=0
  CM2 : powerlib/Measurements/Current Measurement  PhasorSimulation=off  OutputType=Complex  PSBequivalent=0
  CM3 : powerlib/Measurements/Current Measurement  PhasorSimulation=off  OutputType=Complex  PSBequivalent=0
  DC Voltage Source : powerlib/Electrical Sources/DC Voltage Source  Commented=on  Amplitude=Vdc_Bat1  Measurements=None
  P : Product  Commented=on  Inputs=**
  P1 : Product  Commented=on  Inputs=**
  Parallel RLC Branch1 : powerlib/Elements/Parallel RLC Branch  LConnTagsString=a  RConnTagsString=__new0  BranchType=R  Resistance=1500  Inductance=0  SetiL0=off  InitialCurrent=0  Capacitance=Cdc_Bat1  Setx0=on  InitialVoltage=700  Measurements=None
  Parallel RLC Branch2 : powerlib/Elements/Parallel RLC Branch  LConnTagsString=a  RConnTagsString=__new0  BranchType=C  Resistance=10000000  Inductance=0  SetiL0=off  InitialCurrent=0  Capacitance=Cdc_Bat1  Setx0=on  InitialVoltage=700  Measurements=None
  Parallel RLC Branch3 : powerlib/Elements/Parallel RLC Branch  LConnTagsString=a  RConnTagsString=__new0  BranchType=R  Resistance=0.00001  Inductance=0  SetiL0=off  InitialCurrent=0  Capacitance=Cdc_Bat1  Setx0=on  InitialVoltage=700  Measurements=None
  VM1 : powerlib/Measurements/Voltage Measurement  PhasorSimulation=off  OutputType=Complex  PSBequivalent=0
  w1 : Scope  Commented=on
  w2 : Scope  Commented=on
  w3 : Scope  Commented=on  NumInputPorts=2
  w7 : Scope  Commented=on
  + in : PMIOPort  Port=1  Side=Left
  - in : PMIOPort  Port=2  Side=Left
  + out : PMIOPort  Port=3  Side=Right
  - out : PMIOPort  Port=4  Side=Right
  Vdc : Outport
  wires:
  P/1 -> w3/2, w2/1
  CM1/1 -> P/1
  CM2/1 -> w7/1
  P1/1 -> w3/1, w1/1
  CM3/1 -> P1/1
  VM1/1 -> Vdc/1, P1/2, P/2
  connections:
  Parallel RLC Branch2/LConn1 -- CM2/LConn1
  CM2/RConn1 -- Parallel RLC Branch3/LConn1 -- VM1/LConn1 -- CM1/LConn1
  - in/RConn1 -- Parallel RLC Branch1/RConn1 -- - out/RConn1 -- DC Voltage Source/LConn1 -- VM1/LConn2 -- Parallel RLC Branch2/RConn1
  Parallel RLC Branch1/LConn1 -- CM3/LConn1 -- + in/RConn1
  DC Voltage Source/RConn1 -- CM1/RConn1 -- + out/RConn1
  CM3/RConn1 -- Parallel RLC Branch3/RConn1

== system MR_CIGRE_GENERALIZADO/Banco de Baterias_2/Imp. Virtual1 ==
  Id : Inport
  Iq : Inport  Port=2
  W : Inport  Port=3
  HPF1 : TransferFcn  Numerator=[1 0]  Denominator=[1 100]
  HPF2 : TransferFcn  Numerator=[1 0]  Denominator=[1 100]
  Product1 : Product
  Product3 : Product
  Sum1 : Sum  Inputs=|++
  Sum2 : Sum  Inputs=|++
  Sum5 : Sum  Inputs=++|
  Sum6 : Sum  Inputs=++|
  Zvdd : Gain  Gain=L_Virt_Bat2
  Zvdq1 : Gain  Gain=-L_Virt_Bat2
  Zvqd : Gain  Gain=L_Virt_Bat2
  Zvqq : Gain  Gain=L_Virt_Bat2
  Zvqq1 : Gain  Gain=R_Virt_Bat2
  Zvqq2 : Gain  Gain=R_Virt_Bat2
  Vd_Zv : Outport
  Vq_Zv : Outport  Port=2
  wires:
  Zvqd/1 -> Product3/2
  W/1 -> Product1/2, Product3/1
  Sum6/1 -> Vq_Zv/1
  Zvdd/1 -> HPF1/1
  Product1/1 -> Sum5/2
  Zvqq/1 -> HPF2/1
  Id/1 -> Zvqd/1, Zvqq2/1, Zvdd/1
  Product3/1 -> Sum6/1
  Sum5/1 -> Vd_Zv/1
  Zvdq1/1 -> Product1/1
  Iq/1 -> Zvqq1/1, Zvdq1/1, Zvqq/1
  HPF2/1 -> Sum1/1
  Zvqq1/1 -> Sum1/2
  Sum1/1 -> Sum6/2
  HPF1/1 -> Sum2/1
  Zvqq2/1 -> Sum2/2
  Sum2/1 -> Sum5/1

== system MR_CIGRE_GENERALIZADO/Banco de Baterias_2/Inversor CC//CA ==
  Vabc : Inport
  R+ron+L VSC2 : powerlib/Elements/Three-Phase Series RLC Branch  LConnTagsString=A|B|C  RConnTagsString=A|B|C  BranchType=RL  Resistance=R_Bat1+ron_Bat1  Inductance=L_Bat1  Capacitance=1e-6  Measurements=None
  Sequence Analyzer5 : powerlib_meascontrol/Measurements/Sequence Analyzer  Commented=on  Freq=60  n=1  seq=Positive  InInit=[1, 0]  Ts=0
      settings: SourceProductName=Simscape Power Systems  SourceProductBaseCode=PS
  Three-Phase Series RLC Branch1 : powerlib/Elements/Three-Phase Series RLC Branch  LConnTagsString=A|B|C  RConnTagsString=A|B|C  BranchType=C  Resistance=1  Inductance=1e-3  Capacitance=Cf_Bat1  Measurements=None
  V&I - VSC2 2 : powerlib/Measurements/Three-Phase V-I Measurement  VoltageMeasurement=phase-to-ground  SetLabelV=off  LabelV=Vabc  Vpu=off  VpuLL=off  CurrentMeasurement=yes  SetLabelI=off  LabelI=Iabc  Ipu=off  Pbase=100e6  Vbase=500e3  OutputType=Complex  PhasorSimulation=off  PSBequivalent=0
  VSC (Average Model) : powerlib/Power Electronics/Universal Bridge  Arms=3  SnubberResistance=1e5  SnubberCapacitance=inf  Device=Average-model based VSC  Ron=1e-3  Lon=0  ForwardVoltages="[  0  0  ]"  ForwardVoltage=0  GTOparameters=[ 10e-6 , 20e-6 ]  IGBTparameters=[ 1e-6 , 2e-6 ]  Measurements=None  Measurements_2=None  converterType=Rectifier
  w4 : Scope  Commented=on
  Va : PMIOPort  Port=1  Side=Right
  Vb : PMIOPort  Port=2  Side=Right
  Vc : PMIOPort  Port=3  Side=Right
  GND : PMIOPort  Port=4  Side=Right
  + : PMIOPort  Port=5  Side=Left
  - : PMIOPort  Port=6  Side=Left
  Vabc_M : Outport
  Iabc_M : Outport  Port=2
  wires:
  V&I - VSC2 2/2 -> Iabc_M/1
  Sequence Analyzer5/1 -> w4/1
  V&I - VSC2 2/1 -> Vabc_M/1
  Vabc/1 -> Sequence Analyzer5/1, VSC (Average Model)/1
  connections:
  Three-Phase Series RLC Branch1/RConn1 -- Three-Phase Series RLC Branch1/RConn3 -- Three-Phase Series RLC Branch1/RConn2 -- GND/RConn1
  V&I - VSC2 2/RConn1 -- R+ron+L VSC2/LConn1
  V&I - VSC2 2/RConn2 -- R+ron+L VSC2/LConn2
  V&I - VSC2 2/RConn3 -- R+ron+L VSC2/LConn3
  Three-Phase Series RLC Branch1/LConn1 -- Va/RConn1 -- R+ron+L VSC2/RConn1
  Three-Phase Series RLC Branch1/LConn2 -- Vb/RConn1 -- R+ron+L VSC2/RConn2
  Three-Phase Series RLC Branch1/LConn3 -- Vc/RConn1 -- R+ron+L VSC2/RConn3
  VSC (Average Model)/LConn1 -- V&I - VSC2 2/LConn1
  VSC (Average Model)/LConn2 -- V&I - VSC2 2/LConn2
  VSC (Average Model)/LConn3 -- V&I - VSC2 2/LConn3
  VSC (Average Model)/RConn2 -- -/RConn1
  +/RConn1 -- VSC (Average Model)/RConn1

== system MR_CIGRE_GENERALIZADO/Banco de Baterias_2/Medidor de pot ==
  Vd : Inport
  Vq : Inport  Port=2
  Id : Inport  Port=3
  Iq : Inport  Port=4
  Gain : Gain  Gain=1.5
  Gain1 : Gain  Gain=1.5
  Sum1 : Sum  Inputs=+|+
  Sum2 : Sum  Inputs=-|+
  a : Product  Inputs=**
  a1 : Product  Inputs=**
  b1 : Product  Inputs=**
  b2 : Product  Inputs=**
  P : Outport
  Q : Outport  Port=2
  wires:
  a1/1 -> Sum1/2
  Vq/1 -> b2/2, a1/1
  a/1 -> Sum1/1
  b1/1 -> Sum2/1
  Sum1/1 -> Gain/1
  b2/1 -> Sum2/2
  Iq/1 -> b1/2, a1/2
  Vd/1 -> b1/1, a/1
  Id/1 -> b2/1, a/2
  Sum2/1 -> Gain1/1
  Gain/1 -> P/1
  Gain1/1 -> Q/1

== system MR_CIGRE_GENERALIZADO/Banco de Baterias_2/PLL e Medidor1 ==
  note: Medida de w e wt do Sistema
  note: Medida Vd, Vq, Iq e Id
  Iabc_M : Inport
  Iabc_S : Inport  Port=2
  Vabc_S : Inport  Port=3
  wt : Inport  Port=4
  2*pi()*f : Gain  Gain=2*pi()
  Iabc-Idq : powerlib_meascontrol/Transformations/abc to dq0  Alignment=90 degrees behind phase A axis
  Iabc-Idq1 : powerlib_meascontrol/Transformations/abc to dq0  Alignment=90 degrees behind phase A axis
  Iabc-Idq2 : powerlib_meascontrol/Transformations/abc to dq0  Alignment=90 degrees behind phase A axis
  PLL (3ph) : powerlib_meascontrol/PLL/PLL (3ph)  Fmin=1  Par_Init="[0  f0]"  ParK=[180, 3200, 1]  TcD=5E-5  MaxRateChangeFreq=120  FilterCutOffFreq=25  Ts=5E-5  AGC=on
  Sys_wt : Outport
  Sys_w : Outport  Port=2
  Vdq0_S : Outport  Port=3
  Idq_M : Outport  Port=4
  Idq0_S : Outport  Port=5
  wires:
  PLL (3ph)/1 -> 2*pi()*f/1
  Iabc_S/1 -> Iabc-Idq/1
  Vabc_S/1 -> Iabc-Idq1/1, PLL (3ph)/1
  Iabc_M/1 -> Iabc-Idq2/1
  Iabc-Idq/1 -> Idq0_S/1
  Iabc-Idq2/1 -> Idq_M/1
  Iabc-Idq1/1 -> Vdq0_S/1
  2*pi()*f/1 -> Sys_w/1
  wt/1 -> [wt]
  PLL (3ph)/2 -> Sys_wt/1
  [wt] -> Iabc-Idq2/2
  [wt] -> Iabc-Idq/2
  [wt] -> Iabc-Idq1/2

== system MR_CIGRE_GENERALIZADO/Banco de Baterias_2/Referecia Tensao e Freq. angular ==
  Inc_w_pu : Inport
  Inc_E_pu : Inport  Port=2
  Sum1 : Sum  Inputs=+|+
  Sum2 : Sum  Inputs=+|+
  ref : Step  Time=0  SampleTime=0
  ref2 : Step  Time=0  SampleTime=0
  w_ref_pu : Outport
  V_ref_pu : Outport  Port=2
  wires:
  Inc_E_pu/1 -> Sum1/1
  Sum1/1 -> V_ref_pu/1
  Sum2/1 -> w_ref_pu/1
  ref/1 -> Sum2/1
  Inc_w_pu/1 -> Sum2/2
  ref2/1 -> Sum1/2

== system MR_CIGRE_GENERALIZADO/Banco de Baterias_2/Referencia de  Corrente ==
  Id_feed : Inport
  Iq_feed : Inport  Port=2
  Sw_Mode : Inport  Port=3
  Id_supp : Inport  Port=4
  Iq_supp : Inport  Port=5
  LPF2 : TransferFcn  Denominator=[1/(LPF_Cv_Bat1) 1]
  LPF4 : TransferFcn  Denominator=[1/(LPF_Cv_Bat1) 1]
  Switch : Switch  Criteria=u2 > Threshold
  Switch1 : Switch  Criteria=u2 > Threshold
  Id_ref : Outport
  Iq_ref : Outport  Port=2
  wires:
  Sw_Mode/1 -> Switch/2, Switch1/2
  Switch/1 -> LPF4/1
  Switch1/1 -> LPF2/1
  Id_feed/1 -> Switch/1
  Id_supp/1 -> Switch/3
  Iq_feed/1 -> Switch1/1
  Iq_supp/1 -> Switch1/3
  LPF2/1 -> Iq_ref/1
  LPF4/1 -> Id_ref/1

== system MR_CIGRE_GENERALIZADO/Banco de Baterias_2/Referência de Potencia ==
  note: Mudança de referência: no sincronismo (sinc=1)
  note: Ref. Potencia em rampa p.u.
  sinc : Inport
  Pref_bat : Inport  Port=2
  Qref_bat : Inport  Port=3
  Pgd : Inport  Port=4
  Qgd : Inport  Port=5
  Data Store Memory : DataStoreMemory  DataStoreName=Qr  ReadBeforeWriteMsg=warning  WriteAfterWriteMsg=warning  WriteAfterReadMsg=warning  ShowAdditionalParam=off  OutDataTypeStr=double
  Data Store Memory1 : DataStoreMemory  DataStoreName=Pr  ReadBeforeWriteMsg=warning  WriteAfterWriteMsg=warning  WriteAfterReadMsg=warning  VectorParams1D=off  ShowAdditionalParam=off  OutDataTypeStr=double
  Product1 : Product
  Product2 : Product
  Rate Limiter : RateLimiter  RisingSlewLimit=PQ_ref_taxavar_bat1*Sb_Bat1  FallingSlewLimit=-PQ_ref_taxavar_bat1*Sb_Bat1  SampleTimeMode=inherited
  Rate Limiter1 : RateLimiter  RisingSlewLimit=PQ_ref_taxavar_bat1*Sb_Bat1  FallingSlewLimit=-PQ_ref_taxavar_bat1*Sb_Bat1  SampleTimeMode=inherited
  Referência Fonte : MATLAB Function  TreatAsAtomicUnit=on
  Time_init_ref : Step  Time=PQ_ref_time_bat1  SampleTime=0
  Prefbat : Outport
  Qrefbat : Outport  Port=2
  wires:
  Referência Fonte/1(Prefbat) -> Prefbat/1
  Referência Fonte/2(Qrefbat) -> Qrefbat/1
  sinc/1 -> Referência Fonte/5(sinc)
  Pgd/1 -> Referência Fonte/3(p)
  Qgd/1 -> Referência Fonte/4(q)
  Product2/1 -> Rate Limiter1/1
  Time_init_ref/1 -> Product1/2, Product2/1
  Qref_bat/1 -> Product2/2
  Product1/1 -> Rate Limiter/1
  Pref_bat/1 -> Product1/1
  Rate Limiter/1 -> Referência Fonte/1(Pref_bat)
  Rate Limiter1/1 -> Referência Fonte/2(Qref_bat)

== system MR_CIGRE_GENERALIZADO/PCC/Ilhamento// Sincronização ==
  sinc : Inport
  Display : Display
  Display1 : Display
  Display3 : Display
  Ilhamento Chave fechada para chave aberta em tilha : Step  Time=tilha  Before=1  After=0  SampleTime=0
  Switch : Switch  Criteria=u2 > Threshold
  sinc=1 : Constant
  "Ch " : Outport
  wires:
  Ilhamento Chave fechada para chave aberta em tilha/1 -> Switch/3, Display3/1
  sinc=1/1 -> Switch/1, Display/1
  Switch/1 -> "Ch "/1, Display1/1
  sinc/1 -> Switch/2
